simulink model "Gait2392_simbody_simscape"  (R2025b)
(part 2 of 16)

  vas_med_l_vas_med_l_P3_y : sm_lib/Joints/Prismatic Joint  JointMode=Normal  CompositeWrenchDir=FollowerOnBase  CompositeWrenchFrame=BaseFrame  SenseConstraintForce=off  SenseConstraintTorque=off  SenseTotalForce=off  SenseTotalTorque=off  PositionTargetSpecify=off  PositionTargetPriority=High  PositionTargetValue=0  PositionTargetValueUnits=m  VelocityTargetSpecify=off  VelocityTargetPriority=High  VelocityTargetValue=0  VelocityTargetValueUnits=m/s  EquilibriumPosition=0  EquilibriumPositionUnits=m  SpringStiffness=0  SpringStiffnessUnits=N/m  DampingCoefficient=0  DampingCoefficientUnits=kg/s  LowerLimitSpecify=on  LowerLimitBound=-0.4048  LowerLimitBoundUnits=m  LowerLimitStiffness=1e6  LowerLimitStiffnessUnits=N/m  LowerLimitDamping=1e3  LowerLimitDampingUnits=N/(m/s)  LowerLimitTransitionRegionWidth=1e-4  LowerLimitTransitionRegionWidthUnits=m  UpperLimitSpecify=on  UpperLimitBound=-0.2769  UpperLimitBoundUnits=m  UpperLimitStiffness=1e6  UpperLimitStiffnessUnits=N/m  UpperLimitDamping=1e3  UpperLimitDampingUnits=N/(m/s)  UpperLimitTransitionRegionWidth=1e-4  UpperLimitTransitionRegionWidthUnits=m  TorqueActuationMode=NoTorque  MotionActuationMode=ComputedMotion  SensePosition=off  SenseVelocity=off  SenseAcceleration=off  SenseTorqueForce=off  SenseLowerLimitTorqueForce=off  SenseUpperLimitTorqueForce=off
  vas_med_l_vas_med_l_P3_z : sm_lib/Joints/Prismatic Joint  JointMode=Normal  CompositeWrenchDir=FollowerOnBase  CompositeWrenchFrame=BaseFrame  SenseConstraintForce=off  SenseConstraintTorque=off  SenseTotalForce=off  SenseTotalTorque=off  PositionTargetSpecify=off  PositionTargetPriority=High  PositionTargetValue=0  PositionTargetValueUnits=m  VelocityTargetSpecify=off  VelocityTargetPriority=High  VelocityTargetValue=0  VelocityTargetValueUnits=m/s  EquilibriumPosition=0  EquilibriumPositionUnits=m  SpringStiffness=0  SpringStiffnessUnits=N/m  DampingCoefficient=0  DampingCoefficientUnits=kg/s  LowerLimitSpecify=on  LowerLimitBound=-0.0009  LowerLimitBoundUnits=m  LowerLimitStiffness=1e6  LowerLimitStiffnessUnits=N/m  LowerLimitDamping=1e3  LowerLimitDampingUnits=N/(m/s)  LowerLimitTransitionRegionWidth=1e-4  LowerLimitTransitionRegionWidthUnits=m  UpperLimitSpecify=on  UpperLimitBound=0.0125  UpperLimitBoundUnits=m  UpperLimitStiffness=1e6  UpperLimitStiffnessUnits=N/m  UpperLimitDamping=1e3  UpperLimitDampingUnits=N/(m/s)  UpperLimitTransitionRegionWidth=1e-4  UpperLimitTransitionRegionWidthUnits=m  TorqueActuationMode=NoTorque  MotionActuationMode=ComputedMotion  SensePosition=off  SenseVelocity=off  SenseAcceleration=off  SenseTorqueForce=off  SenseLowerLimitTorqueForce=off  SenseUpperLimitTorqueForce=off
  vas_med_l_vas_med_l_P4 : Subsystem
  vas_med_l_vas_med_l_P4_frame_fix : sm_lib/Joints/Weld Joint  JointMode=Normal  CompositeWrenchDir=FollowerOnBase  CompositeWrenchFrame=BaseFrame  SenseConstraintForce=off  SenseConstraintTorque=off  SenseTotalForce=off  SenseTotalTorque=off
  vas_med_l_vas_med_l_P4_vas_med_l_vas_med_l_P4_x_f : Subsystem
  vas_med_l_vas_med_l_P4_vas_med_l_vas_med_l_P4_y_f : Subsystem
  vas_med_l_vas_med_l_P4_vas_med_l_vas_med_l_P4_z_f : Subsystem
  vas_med_l_vas_med_l_P4_x : sm_lib/Joints/Prismatic Joint  JointMode=Normal  CompositeWrenchDir=FollowerOnBase  CompositeWrenchFrame=BaseFrame  SenseConstraintForce=off  SenseConstraintTorque=off  SenseTotalForce=off  SenseTotalTorque=off  PositionTargetSpecify=off  PositionTargetPriority=High  PositionTargetValue=0  PositionTargetValueUnits=m  VelocityTargetSpecify=off  VelocityTargetPriority=High  VelocityTargetValue=0  VelocityTargetValueUnits=m/s  EquilibriumPosition=0  EquilibriumPositionUnits=m  SpringStiffness=0  SpringStiffnessUnits=N/m  DampingCoefficient=0  DampingCoefficientUnits=kg/s  LowerLimitSpecify=on  LowerLimitBound=0.0274  LowerLimitBoundUnits=m  LowerLimitStiffness=1e6  LowerLimitStiffnessUnits=N/m  LowerLimitDamping=1e3  LowerLimitDampingUnits=N/(m/s)  LowerLimitTransitionRegionWidth=1e-4  LowerLimitTransitionRegionWidthUnits=m  UpperLimitSpecify=on  UpperLimitBound=0.0356  UpperLimitBoundUnits=m  UpperLimitStiffness=1e6  UpperLimitStiffnessUnits=N/m  UpperLimitDamping=1e3  UpperLimitDampingUnits=N/(m/s)  UpperLimitTransitionRegionWidth=1e-4  UpperLimitTransitionRegionWidthUnits=m  TorqueActuationMode=NoTorque  MotionActuationMode=ComputedMotion  SensePosition=off  SenseVelocity=off  SenseAcceleration=off  SenseTorqueForce=off  SenseLowerLimitTorqueForce=off  SenseUpperLimitTorqueForce=off
  vas_med_l_vas_med_l_P4_y : sm_lib/Joints/Prismatic Joint  JointMode=Normal  CompositeWrenchDir=FollowerOnBase  CompositeWrenchFrame=BaseFrame  SenseConstraintForce=off  SenseConstraintTorque=off  SenseTotalForce=off  SenseTotalTorque=off  PositionTargetSpecify=off  PositionTargetPriority=High  PositionTargetValue=0  PositionTargetValueUnits=m  VelocityTargetSpecify=off  VelocityTargetPriority=High  VelocityTargetValue=0  VelocityTargetValueUnits=m/s  EquilibriumPosition=0  EquilibriumPositionUnits=m  SpringStiffness=0  SpringStiffnessUnits=N/m  DampingCoefficient=0  DampingCoefficientUnits=kg/s  LowerLimitSpecify=on  LowerLimitBound=-0.4255  LowerLimitBoundUnits=m  LowerLimitStiffness=1e6  LowerLimitStiffnessUnits=N/m  LowerLimitDamping=1e3  LowerLimitDampingUnits=N/(m/s)  LowerLimitTransitionRegionWidth=1e-4  LowerLimitTransitionRegionWidthUnits=m  UpperLimitSpecify=on  UpperLimitBound=-0.2769  UpperLimitBoundUnits=m  UpperLimitStiffness=1e6  UpperLimitStiffnessUnits=N/m  UpperLimitDamping=1e3  UpperLimitDampingUnits=N/(m/s)  UpperLimitTransitionRegionWidth=1e-4  UpperLimitTransitionRegionWidthUnits=m  TorqueActuationMode=NoTorque  MotionActuationMode=ComputedMotion  SensePosition=off  SenseVelocity=off  SenseAcceleration=off  SenseTorqueForce=off  SenseLowerLimitTorqueForce=off  SenseUpperLimitTorqueForce=off
  vas_med_l_vas_med_l_P4_z : sm_lib/Joints/Prismatic Joint  JointMode=Normal  CompositeWrenchDir=FollowerOnBase  CompositeWrenchFrame=BaseFrame  SenseConstraintForce=off  SenseConstraintTorque=off  SenseTotalForce=off  SenseTotalTorque=off  PositionTargetSpecify=off  PositionTargetPriority=High  PositionTargetValue=0  PositionTargetValueUnits=m  VelocityTargetSpecify=off  VelocityTargetPriority=High  VelocityTargetValue=0  VelocityTargetValueUnits=m/s  EquilibriumPosition=0  EquilibriumPositionUnits=m  SpringStiffness=0  SpringStiffnessUnits=N/m  DampingCoefficient=0  DampingCoefficientUnits=kg/s  LowerLimitSpecify=on  LowerLimitBound=-0.0009  LowerLimitBoundUnits=m  LowerLimitStiffness=1e6  LowerLimitStiffnessUnits=N/m  LowerLimitDamping=1e3  LowerLimitDampingUnits=N/(m/s)  LowerLimitTransitionRegionWidth=1e-4  LowerLimitTransitionRegionWidthUnits=m  UpperLimitSpecify=on  UpperLimitBound=0.0131  UpperLimitBoundUnits=m  UpperLimitStiffness=1e6  UpperLimitStiffnessUnits=N/m  UpperLimitDamping=1e3  UpperLimitDampingUnits=N/(m/s)  UpperLimitTransitionRegionWidth=1e-4  UpperLimitTransitionRegionWidthUnits=m  TorqueActuationMode=NoTorque  MotionActuationMode=ComputedMotion  SensePosition=off  SenseVelocity=off  SenseAcceleration=off  SenseTorqueForce=off  SenseLowerLimitTorqueForce=off  SenseUpperLimitTorqueForce=off
  vas_med_l_vas_med_l_P5 : Subsystem
  vas_med_l_vas_med_l_P5_frame_fix : sm_lib/Joints/Weld Joint  JointMode=Normal  CompositeWrenchDir=FollowerOnBase  CompositeWrenchFrame=BaseFrame  SenseConstraintForce=off  SenseConstraintTorque=off  SenseTotalForce=off  SenseTotalTorque=off
  vas_med_l_vas_med_l_P5_vas_med_l_vas_med_l_P5_x_f : Subsystem
  vas_med_l_vas_med_l_P5_vas_med_l_vas_med_l_P5_y_f : Subsystem
  vas_med_l_vas_med_l_P5_x : sm_lib/Joints/Prismatic Joint  JointMode=Normal  CompositeWrenchDir=FollowerOnBase  CompositeWrenchFrame=BaseFrame  SenseConstraintForce=off  SenseConstraintTorque=off  SenseTotalForce=off  SenseTotalTorque=off  PositionTargetSpecify=off  PositionTargetPriority=High  PositionTargetValue=0  PositionTargetValueUnits=m  VelocityTargetSpecify=off  VelocityTargetPriority=High  VelocityTargetValue=0  VelocityTargetValueUnits=m/s  EquilibriumPosition=0  EquilibriumPositionUnits=m  SpringStiffness=0  SpringStiffnessUnits=N/m  DampingCoefficient=0  DampingCoefficientUnits=kg/s  LowerLimitSpecify=on  LowerLimitBound=0.009811  LowerLimitBoundUnits=m  LowerLimitStiffness=1e6  LowerLimitStiffnessUnits=N/m  LowerLimitDamping=1e3  LowerLimitDampingUnits=N/(m/s)  LowerLimitTransitionRegionWidth=1e-4  LowerLimitTransitionRegionWidthUnits=m  UpperLimitSpecify=on  UpperLimitBound=0.06795  UpperLimitBoundUnits=m  UpperLimitStiffness=1e6  UpperLimitStiffnessUnits=N/m  UpperLimitDamping=1e3  UpperLimitDampingUnits=N/(m/s)  UpperLimitTransitionRegionWidth=1e-4  UpperLimitTransitionRegionWidthUnits=m  TorqueActuationMode=NoTorque  MotionActuationMode=ComputedMotion  SensePosition=off  SenseVelocity=off  SenseAcceleration=off  SenseTorqueForce=off  SenseLowerLimitTorqueForce=off  SenseUpperLimitTorqueForce=off
  vas_med_l_vas_med_l_P5_y : sm_lib/Joints/Prismatic Joint  JointMode=Normal  CompositeWrenchDir=FollowerOnBase  CompositeWrenchFrame=BaseFrame  SenseConstraintForce=off  SenseConstraintTorque=off  SenseTotalForce=off  SenseTotalTorque=off  PositionTargetSpecify=off  PositionTargetPriority=High  PositionTargetValue=0  PositionTargetValueUnits=m  VelocityTargetSpecify=off  VelocityTargetPriority=High  VelocityTargetValue=0  VelocityTargetValueUnits=m/s  EquilibriumPosition=0  EquilibriumPositionUnits=m  SpringStiffness=0  SpringStiffnessUnits=N/m  DampingCoefficient=0  DampingCoefficientUnits=kg/s  LowerLimitSpecify=on  LowerLimitBound=-0.06562  LowerLimitBoundUnits=m  LowerLimitStiffness=1e6  LowerLimitStiffnessUnits=N/m  LowerLimitDamping=1e3  LowerLimitDampingUnits=N/(m/s)  LowerLimitTransitionRegionWidth=1e-4  LowerLimitTransitionRegionWidthUnits=m  UpperLimitSpecify=on  UpperLimitBound=0.02433  UpperLimitBoundUnits=m  UpperLimitStiffness=1e6  UpperLimitStiffnessUnits=N/m  UpperLimitDamping=1e3  UpperLimitDampingUnits=N/(m/s)  UpperLimitTransitionRegionWidth=1e-4  UpperLimitTransitionRegionWidthUnits=m  TorqueActuationMode=NoTorque  MotionActuationMode=ComputedMotion  SensePosition=off  SenseVelocity=off  SenseAcceleration=off  SenseTorqueForce=off  SenseLowerLimitTorqueForce=off  SenseUpperLimitTorqueForce=off
  vas_med_r_vas_med_r_P3 : Subsystem
  vas_med_r_vas_med_r_P3_frame_fix : sm_lib/Joints/Weld Joint  JointMode=Normal  CompositeWrenchDir=FollowerOnBase  CompositeWrenchFrame=BaseFrame  SenseConstraintForce=off  SenseConstraintTorque=off  SenseTotalForce=off  SenseTotalTorque=off
  vas_med_r_vas_med_r_P3_vas_med_r_vas_med_r_P3_x_f : Subsystem
  vas_med_r_vas_med_r_P3_vas_med_r_vas_med_r_P3_y_f : Subsystem
  vas_med_r_vas_med_r_P3_vas_med_r_vas_med_r_P3_z_f : Subsystem
  vas_med_r_vas_med_r_P3_x : sm_lib/Joints/Prismatic Joint  JointMode=Normal  CompositeWrenchDir=FollowerOnBase  CompositeWrenchFrame=BaseFrame  SenseConstraintForce=off  SenseConstraintTorque=off  SenseTotalForce=off  SenseTotalTorque=off  PositionTargetSpecify=off  PositionTargetPriority=High  PositionTargetValue=0  PositionTargetValueUnits=m  VelocityTargetSpecify=off  VelocityTargetPriority=High  VelocityTargetValue=0  VelocityTargetValueUnits=m/s  EquilibriumPosition=0  EquilibriumPositionUnits=m  SpringStiffness=0  SpringStiffnessUnits=N/m  DampingCoefficient=0  DampingCoefficientUnits=kg/s  LowerLimitSpecify=on  LowerLimitBound=0.0356  LowerLimitBoundUnits=m  LowerLimitStiffness=1e6  LowerLimitStiffnessUnits=N/m  LowerLimitDamping=1e3  LowerLimitDampingUnits=N/(m/s)  LowerLimitTransitionRegionWidth=1e-4  LowerLimitTransitionRegionWidthUnits=m  UpperLimitSpecify=on  UpperLimitBound=0.037  UpperLimitBoundUnits=m  UpperLimitStiffness=1e6  UpperLimitStiffnessUnits=N/m  UpperLimitDamping=1e3  UpperLimitDampingUnits=N/(m/s)  UpperLimitTransitionRegionWidth=1e-4  UpperLimitTransitionRegionWidthUnits=m  TorqueActuationMode=NoTorque  MotionActuationMode=ComputedMotion  SensePosition=off  SenseVelocity=off  SenseAcceleration=off  SenseTorqueForce=off  SenseLowerLimitTorqueForce=off  SenseUpperLimitTorqueForce=off
  vas_med_r_vas_med_r_P3_y : sm_lib/Joints/Prismatic Joint  JointMode=Normal  CompositeWrenchDir=FollowerOnBase  CompositeWrenchFrame=BaseFrame  SenseConstraintForce=off  SenseConstraintTorque=off  SenseTotalForce=off  SenseTotalTorque=off  PositionTargetSpecify=off  PositionTargetPriority=High  PositionTargetValue=0  PositionTargetValueUnits=m  VelocityTargetSpecify=off  VelocityTargetPriority=High  VelocityTargetValue=0  VelocityTargetValueUnits=m/s  EquilibriumPosition=0  EquilibriumPositionUnits=m  SpringStiffness=0  SpringStiffnessUnits=N/m  DampingCoefficient=0  DampingCoefficientUnits=kg/s  LowerLimitSpecify=on  LowerLimitBound=-0.4048  LowerLimitBoundUnits=m  LowerLimitStiffness=1e6  LowerLimitStiffnessUnits=N/m  LowerLimitDamping=1e3  LowerLimitDampingUnits=N/(m/s)  LowerLimitTransitionRegionWidth=1e-4  LowerLimitTransitionRegionWidthUnits=m  UpperLimitSpecify=on  UpperLimitBound=-0.2769  UpperLimitBoundUnits=m  UpperLimitStiffness=1e6  UpperLimitStiffnessUnits=N/m  UpperLimitDamping=1e3  UpperLimitDampingUnits=N/(m/s)  UpperLimitTransitionRegionWidth=1e-4  UpperLimitTransitionRegionWidthUnits=m  TorqueActuationMode=NoTorque  MotionActuationMode=ComputedMotion  SensePosition=off  SenseVelocity=off  SenseAcceleration=off  SenseTorqueForce=off  SenseLowerLimitTorqueForce=off  SenseUpperLimitTorqueForce=off
  vas_med_r_vas_med_r_P3_z : sm_lib/Joints/Prismatic Joint  JointMode=Normal  CompositeWrenchDir=FollowerOnBase  CompositeWrenchFrame=BaseFrame  SenseConstraintForce=off  SenseConstraintTorque=off  SenseTotalForce=off  SenseTotalTorque=off  PositionTargetSpecify=off  PositionTargetPriority=High  PositionTargetValue=0  PositionTargetValueUnits=m  VelocityTargetSpecify=off  VelocityTargetPriority=High  VelocityTargetValue=0  VelocityTargetValueUnits=m/s  EquilibriumPosition=0  EquilibriumPositionUnits=m  SpringStiffness=0  SpringStiffnessUnits=N/m  DampingCoefficient=0  DampingCoefficientUnits=kg/s  LowerLimitSpecify=on  LowerLimitBound=-0.0125  LowerLimitBoundUnits=m  LowerLimitStiffness=1e6  LowerLimitStiffnessUnits=N/m  LowerLimitDamping=1e3  LowerLimitDampingUnits=N/(m/s)  LowerLimitTransitionRegionWidth=1e-4  LowerLimitTransitionRegionWidthUnits=m  UpperLimitSpecify=on  UpperLimitBound=0.0009  UpperLimitBoundUnits=m  UpperLimitStiffness=1e6  UpperLimitStiffnessUnits=N/m  UpperLimitDamping=1e3  UpperLimitDampingUnits=N/(m/s)  UpperLimitTransitionRegionWidth=1e-4  UpperLimitTransitionRegionWidthUnits=m  TorqueActuationMode=NoTorque  MotionActuationMode=ComputedMotion  SensePosition=off  SenseVelocity=off  SenseAcceleration=off  SenseTorqueForce=off  SenseLowerLimitTorqueForce=off  SenseUpperLimitTorqueForce=off
  vas_med_r_vas_med_r_P4 : Subsystem
  vas_med_r_vas_med_r_P4_frame_fix : sm_lib/Joints/Weld Joint  JointMode=Normal  CompositeWrenchDir=FollowerOnBase  CompositeWrenchFrame=BaseFrame  SenseConstraintForce=off  SenseConstraintTorque=off  SenseTotalForce=off  SenseTotalTorque=off
  vas_med_r_vas_med_r_P4_vas_med_r_vas_med_r_P4_x_f : Subsystem
  vas_med_r_vas_med_r_P4_vas_med_r_vas_med_r_P4_y_f : Subsystem
  vas_med_r_vas_med_r_P4_vas_med_r_vas_med_r_P4_z_f : Subsystem
  vas_med_r_vas_med_r_P4_x : sm_lib/Joints/Prismatic Joint  JointMode=Normal  CompositeWrenchDir=FollowerOnBase  CompositeWrenchFrame=BaseFrame  SenseConstraintForce=off  SenseConstraintTorque=off  SenseTotalForce=off  SenseTotalTorque=off  PositionTargetSpecify=off  PositionTargetPriority=High  PositionTargetValue=0  PositionTargetValueUnits=m  VelocityTargetSpecify=off  VelocityTargetPriority=High  VelocityTargetValue=0  VelocityTargetValueUnits=m/s  EquilibriumPosition=0  EquilibriumPositionUnits=m  SpringStiffness=0  SpringStiffnessUnits=N/m  DampingCoefficient=0  DampingCoefficientUnits=kg/s  LowerLimitSpecify=on  LowerLimitBound=0.0274  LowerLimitBoundUnits=m  LowerLimitStiffness=1e6  LowerLimitStiffnessUnits=N/m  LowerLimitDamping=1e3  LowerLimitDampingUnits=N/(m/s)  LowerLimitTransitionRegionWidth=1e-4  LowerLimitTransitionRegionWidthUnits=m  UpperLimitSpecify=on  UpperLimitBound=0.0356  UpperLimitBoundUnits=m  UpperLimitStiffness=1e6  UpperLimitStiffnessUnits=N/m  UpperLimitDamping=1e3  UpperLimitDampingUnits=N/(m/s)  UpperLimitTransitionRegionWidth=1e-4  UpperLimitTransitionRegionWidthUnits=m  TorqueActuationMode=NoTorque  MotionActuationMode=ComputedMotion  SensePosition=off  SenseVelocity=off  SenseAcceleration=off  SenseTorqueForce=off  SenseLowerLimitTorqueForce=off  SenseUpperLimitTorqueForce=off
  vas_med_r_vas_med_r_P4_y : sm_lib/Joints/Prismatic Joint  JointMode=Normal  CompositeWrenchDir=FollowerOnBase  CompositeWrenchFrame=BaseFrame  SenseConstraintForce=off  SenseConstraintTorque=off  SenseTotalForce=off  SenseTotalTorque=off  PositionTargetSpecify=off  PositionTargetPriority=High  PositionTargetValue=0  PositionTargetValueUnits=m  VelocityTargetSpecify=off  VelocityTargetPriority=High  VelocityTargetValue=0  VelocityTargetValueUnits=m/s  EquilibriumPosition=0  EquilibriumPositionUnits=m  SpringStiffness=0  SpringStiffnessUnits=N/m  DampingCoefficient=0  DampingCoefficientUnits=kg/s  LowerLimitSpecify=on  LowerLimitBound=-0.4255  LowerLimitBoundUnits=m  LowerLimitStiffness=1e6  LowerLimitStiffnessUnits=N/m  LowerLimitDamping=1e3  LowerLimitDampingUnits=N/(m/s)  LowerLimitTransitionRegionWidth=1e-4  LowerLimitTransitionRegionWidthUnits=m  UpperLimitSpecify=on  UpperLimitBound=-0.2769  UpperLimitBoundUnits=m  UpperLimitStiffness=1e6  UpperLimitStiffnessUnits=N/m  UpperLimitDamping=1e3  UpperLimitDampingUnits=N/(m/s)  UpperLimitTransitionRegionWidth=1e-4  UpperLimitTransitionRegionWidthUnits=m  TorqueActuationMode=NoTorque  MotionActuationMode=ComputedMotion  SensePosition=off  SenseVelocity=off  SenseAcceleration=off  SenseTorqueForce=off  SenseLowerLimitTorqueForce=off  SenseUpperLimitTorqueForce=off
  vas_med_r_vas_med_r_P4_z : sm_lib/Joints/Prismatic Joint  JointMode=Normal  CompositeWrenchDir=FollowerOnBase  CompositeWrenchFrame=BaseFrame  SenseConstraintForce=off  SenseConstraintTorque=off  SenseTotalForce=off  SenseTotalTorque=off  PositionTargetSpecify=off  PositionTargetPriority=High  PositionTargetValue=0  PositionTargetValueUnits=m  VelocityTargetSpecify=off  VelocityTargetPriority=High  VelocityTargetValue=0  VelocityTargetValueUnits=m/s  EquilibriumPosition=0  EquilibriumPositionUnits=m  SpringStiffness=0  SpringStiffnessUnits=N/m  DampingCoefficient=0  DampingCoefficientUnits=kg/s  LowerLimitSpecify=on  LowerLimitBound=-0.0131  LowerLimitBoundUnits=m  LowerLimitStiffness=1e6  LowerLimitStiffnessUnits=N/m  LowerLimitDamping=1e3  LowerLimitDampingUnits=N/(m/s)  LowerLimitTransitionRegionWidth=1e-4  LowerLimitTransitionRegionWidthUnits=m  UpperLimitSpecify=on  UpperLimitBound=0.0009  UpperLimitBoundUnits=m  UpperLimitStiffness=1e6  UpperLimitStiffnessUnits=N/m  UpperLimitDamping=1e3  UpperLimitDampingUnits=N/(m/s)  UpperLimitTransitionRegionWidth=1e-4  UpperLimitTransitionRegionWidthUnits=m  TorqueActuationMode=NoTorque  MotionActuationMode=ComputedMotion  SensePosition=off  SenseVelocity=off  SenseAcceleration=off  SenseTorqueForce=off  SenseLowerLimitTorqueForce=off  SenseUpperLimitTorqueForce=off
  vas_med_r_vas_med_r_P5 : Subsystem
  vas_med_r_vas_med_r_P5_frame_fix : sm_lib/Joints/Weld Joint  JointMode=Normal  CompositeWrenchDir=FollowerOnBase  CompositeWrenchFrame=BaseFrame  SenseConstraintForce=off  SenseConstraintTorque=off  SenseTotalForce=off  SenseTotalTorque=off
  vas_med_r_vas_med_r_P5_vas_med_r_vas_med_r_P5_x_f : Subsystem
  vas_med_r_vas_med_r_P5_vas_med_r_vas_med_r_P5_y_f : Subsystem
  vas_med_r_vas_med_r_P5_x : sm_lib/Joints/Prismatic Joint  JointMode=Normal  CompositeWrenchDir=FollowerOnBase  CompositeWrenchFrame=BaseFrame  SenseConstraintForce=off  SenseConstraintTorque=off  SenseTotalForce=off  SenseTotalTorque=off  PositionTargetSpecify=off  PositionTargetPriority=High  PositionTargetValue=0  PositionTargetValueUnits=m  VelocityTargetSpecify=off  VelocityTargetPriority=High  VelocityTargetValue=0  VelocityTargetValueUnits=m/s  EquilibriumPosition=0  EquilibriumPositionUnits=m  SpringStiffness=0  SpringStiffnessUnits=N/m  DampingCoefficient=0  DampingCoefficientUnits=kg/s  LowerLimitSpecify=on  LowerLimitBound=0.009811  LowerLimitBoundUnits=m  LowerLimitStiffness=1e6  LowerLimitStiffnessUnits=N/m  LowerLimitDamping=1e3  LowerLimitDampingUnits=N/(m/s)  LowerLimitTransitionRegionWidth=1e-4  LowerLimitTransitionRegionWidthUnits=m  UpperLimitSpecify=on  UpperLimitBound=0.06795  UpperLimitBoundUnits=m  UpperLimitStiffness=1e6  UpperLimitStiffnessUnits=N/m  UpperLimitDamping=1e3  UpperLimitDampingUnits=N/(m/s)  UpperLimitTransitionRegionWidth=1e-4  UpperLimitTransitionRegionWidthUnits=m  TorqueActuationMode=NoTorque  MotionActuationMode=ComputedMotion  SensePosition=off  SenseVelocity=off  SenseAcceleration=off  SenseTorqueForce=off  SenseLowerLimitTorqueForce=off  SenseUpperLimitTorqueForce=off
  vas_med_r_vas_med_r_P5_y : sm_lib/Joints/Prismatic Joint  JointMode=Normal  CompositeWrenchDir=FollowerOnBase  CompositeWrenchFrame=BaseFrame  SenseConstraintForce=off  SenseConstraintTorque=off  SenseTotalForce=off  SenseTotalTorque=off  PositionTargetSpecify=off  PositionTargetPriority=High  PositionTargetValue=0  PositionTargetValueUnits=m  VelocityTargetSpecify=off  VelocityTargetPriority=High  VelocityTargetValue=0  VelocityTargetValueUnits=m/s  EquilibriumPosition=0  EquilibriumPositionUnits=m  SpringStiffness=0  SpringStiffnessUnits=N/m  DampingCoefficient=0  DampingCoefficientUnits=kg/s  LowerLimitSpecify=on  LowerLimitBound=-0.06562  LowerLimitBoundUnits=m  LowerLimitStiffness=1e6  LowerLimitStiffnessUnits=N/m  LowerLimitDamping=1e3  LowerLimitDampingUnits=N/(m/s)  LowerLimitTransitionRegionWidth=1e-4  LowerLimitTransitionRegionWidthUnits=m  UpperLimitSpecify=on  UpperLimitBound=0.02433  UpperLimitBoundUnits=m  UpperLimitStiffness=1e6  UpperLimitStiffnessUnits=N/m  UpperLimitDamping=1e3  UpperLimitDampingUnits=N/(m/s)  UpperLimitTransitionRegionWidth=1e-4  UpperLimitTransitionRegionWidthUnits=m  TorqueActuationMode=NoTorque  MotionActuationMode=ComputedMotion  SensePosition=off  SenseVelocity=off  SenseAcceleration=off  SenseTorqueForce=off  SenseLowerLimitTorqueForce=off  SenseUpperLimitTorqueForce=off
  world : Subsystem
  connections:
  calcn_l/LConn1 -- calcn_l_frame_fix/RConn1
  calcn_l/RConn1 -- mtp_angle_l/LConn1
  femur_l/RConn7 -- lat_gas_l_lat_gas_l_P2_x/LConn1
  pelvis_pelvis_tx_f/LConn1 -- pelvis_tx/RConn1
  pelvis_pelvis_tx_f/RConn1 -- pelvis_ty/LConn1
  pelvis_pelvis_ty_f/LConn1 -- pelvis_ty/RConn1
  pelvis_pelvis_ty_f/RConn1 -- pelvis_tz/LConn1
  pelvis_pelvis_tz_f/LConn1 -- pelvis_tz/RConn1
  pelvis_pelvis_tz_f/RConn1 -- pelvis_tilt/LConn1
  psoas_l_psoas_l_P3/LConn1 -- psoas_l_psoas_l_P3_frame_fix/RConn1
  psoas_l_psoas_l_P3_psoas_l_psoas_l_P3_x_f/LConn1 -- psoas_l_psoas_l_P3_x/RConn1
  psoas_l_psoas_l_P3_psoas_l_psoas_l_P3_x_f/RConn1 -- psoas_l_psoas_l_P3_y/LConn1
  psoas_l_psoas_l_P3_psoas_l_psoas_l_P3_y_f/LConn1 -- psoas_l_psoas_l_P3_y/RConn1
  femur_l/RConn6 -- med_gas_l_med_gas_l_P2_x/LConn1
  psoas_l_psoas_l_P3_psoas_l_psoas_l_P3_y_f/RConn1 -- psoas_l_psoas_l_P3_z/LConn1
  psoas_l_psoas_l_P3_psoas_l_psoas_l_P3_z_f/LConn1 -- psoas_l_psoas_l_P3_z/RConn1
  psoas_l_psoas_l_P3_frame_fix/LConn1 -- psoas_l_psoas_l_P3_psoas_l_psoas_l_P3_z_f/RConn1
  psoas_r_psoas_r_P3/LConn1 -- psoas_r_psoas_r_P3_frame_fix/RConn1
  psoas_r_psoas_r_P3_psoas_r_psoas_r_P3_x_f/LConn1 -- psoas_r_psoas_r_P3_x/RConn1
  psoas_r_psoas_r_P3_psoas_r_psoas_r_P3_x_f/RConn1 -- psoas_r_psoas_r_P3_y/LConn1
  psoas_r_psoas_r_P3_psoas_r_psoas_r_P3_y_f/LConn1 -- psoas_r_psoas_r_P3_y/RConn1
  psoas_r_psoas_r_P3_psoas_r_psoas_r_P3_y_f/RConn1 -- psoas_r_psoas_r_P3_z/LConn1
  psoas_r_psoas_r_P3_psoas_r_psoas_r_P3_z_f/LConn1 -- psoas_r_psoas_r_P3_z/RConn1
  psoas_r_psoas_r_P3_frame_fix/LConn1 -- psoas_r_psoas_r_P3_psoas_r_psoas_r_P3_z_f/RConn1
  femur_l/RConn5 -- vas_int_l_vas_int_l_P3_y/LConn1
  rect_fem_l_rect_fem_l_P3/LConn1 -- rect_fem_l_rect_fem_l_P3_frame_fix/RConn1
  rect_fem_l_rect_fem_l_P3_rect_fem_l_rect_fem_l_P3_x_f/LConn1 -- rect_fem_l_rect_fem_l_P3_x/RConn1
  rect_fem_l_rect_fem_l_P3_rect_fem_l_rect_fem_l_P3_x_f/RConn1 -- rect_fem_l_rect_fem_l_P3_y/LConn1
  rect_fem_l_rect_fem_l_P3_rect_fem_l_rect_fem_l_P3_y_f/LConn1 -- rect_fem_l_rect_fem_l_P3_y/RConn1
  rect_fem_l_rect_fem_l_P3_frame_fix/LConn1 -- rect_fem_l_rect_fem_l_P3_rect_fem_l_rect_fem_l_P3_y_f/RConn1
  rect_fem_r_rect_fem_r_P3/LConn1 -- rect_fem_r_rect_fem_r_P3_frame_fix/RConn1
  rect_fem_r_rect_fem_r_P3_rect_fem_r_rect_fem_r_P3_x_f/LConn1 -- rect_fem_r_rect_fem_r_P3_x/RConn1
  rect_fem_r_rect_fem_r_P3_rect_fem_r_rect_fem_r_P3_x_f/RConn1 -- rect_fem_r_rect_fem_r_P3_y/LConn1
  rect_fem_r_rect_fem_r_P3_rect_fem_r_rect_fem_r_P3_y_f/LConn1 -- rect_fem_r_rect_fem_r_P3_y/RConn1
  rect_fem_r_rect_fem_r_P3_frame_fix/LConn1 -- rect_fem_r_rect_fem_r_P3_rect_fem_r_rect_fem_r_P3_y_f/RConn1
  femur_l/RConn4 -- vas_lat_l_vas_lat_l_P3_x/LConn1
  semimem_l_semimem_l_P2/LConn1 -- semimem_l_semimem_l_P2_frame_fix/RConn1
  semimem_l_semimem_l_P2_semimem_l_semimem_l_P2_x_f/LConn1 -- semimem_l_semimem_l_P2_x/RConn1
  semimem_l_semimem_l_P2_semimem_l_semimem_l_P2_x_f/RConn1 -- semimem_l_semimem_l_P2_y/LConn1
  semimem_l_semimem_l_P2_semimem_l_semimem_l_P2_y_f/LConn1 -- semimem_l_semimem_l_P2_y/RConn1
  semimem_l_semimem_l_P2_frame_fix/LConn1 -- semimem_l_semimem_l_P2_semimem_l_semimem_l_P2_y_f/RConn1
  semimem_r_semimem_r_P2/LConn1 -- semimem_r_semimem_r_P2_frame_fix/RConn1
  semimem_r_semimem_r_P2_semimem_r_semimem_r_P2_x_f/LConn1 -- semimem_r_semimem_r_P2_x/RConn1
  semimem_r_semimem_r_P2_semimem_r_semimem_r_P2_x_f/RConn1 -- semimem_r_semimem_r_P2_y/LConn1
  semimem_r_semimem_r_P2_semimem_r_semimem_r_P2_y_f/LConn1 -- semimem_r_semimem_r_P2_y/RConn1
  semimem_r_semimem_r_P2_frame_fix/LConn1 -- semimem_r_semimem_r_P2_semimem_r_semimem_r_P2_y_f/RConn1
  femur_l/RConn3 -- vas_lat_l_vas_lat_l_P4_x/LConn1
  semiten_l_semiten_l_P2/LConn1 -- semiten_l_semiten_l_P2_frame_fix/RConn1
  semiten_l_semiten_l_P2_semiten_l_semiten_l_P2_x_f/LConn1 -- semiten_l_semiten_l_P2_x/RConn1
  semiten_l_semiten_l_P2_semiten_l_semiten_l_P2_x_f/RConn1 -- semiten_l_semiten_l_P2_y/LConn1
  semiten_l_semiten_l_P2_semiten_l_semiten_l_P2_y_f/LConn1 -- semiten_l_semiten_l_P2_y/RConn1
  semiten_l_semiten_l_P2_frame_fix/LConn1 -- semiten_l_semiten_l_P2_semiten_l_semiten_l_P2_y_f/RConn1
  semiten_r_semiten_r_P2/LConn1 -- semiten_r_semiten_r_P2_frame_fix/RConn1
  semiten_r_semiten_r_P2_semiten_r_semiten_r_P2_x_f/LConn1 -- semiten_r_semiten_r_P2_x/RConn1
  semiten_r_semiten_r_P2_semiten_r_semiten_r_P2_x_f/RConn1 -- semiten_r_semiten_r_P2_y/LConn1
  semiten_r_semiten_r_P2_semiten_r_semiten_r_P2_y_f/LConn1 -- semiten_r_semiten_r_P2_y/RConn1
  semiten_r_semiten_r_P2_frame_fix/LConn1 -- semiten_r_semiten_r_P2_semiten_r_semiten_r_P2_y_f/RConn1
  femur_l/RConn2 -- vas_med_l_vas_med_l_P3_x/LConn1
  talus_l/LConn1 -- talus_l_frame_fix/RConn1
  subtalar_angle_l/LConn1 -- talus_l/RConn1
  ankle_angle_l/RConn1 -- talus_l_ankle_angle_l_f/LConn1
  talus_l_ankle_angle_l_f/RConn1 -- talus_l_frame_fix/LConn1
  talus_r/LConn1 -- talus_r_frame_fix/RConn1
  subtalar_angle_r/LConn1 -- talus_r/RConn1
  ankle_angle_r/RConn1 -- talus_r_ankle_angle_r_f/LConn1
  talus_r_ankle_angle_r_f/RConn1 -- talus_r_frame_fix/LConn1
  tibia_l/LConn1 -- tibia_l_frame_fix/RConn1
  ankle_angle_l/LConn1 -- tibia_l/RConn8
  femur_l/RConn1 -- vas_med_l_vas_med_l_P4_x/LConn1
  grac_l_grac_l_P2_x/LConn1 -- tibia_l/RConn7
  rect_fem_l_rect_fem_l_P3_x/LConn1 -- tibia_l/RConn6
  semimem_l_semimem_l_P2_x/LConn1 -- tibia_l/RConn5
  semiten_l_semiten_l_P2_x/LConn1 -- tibia_l/RConn4
  tibia_l/RConn3 -- vas_int_l_vas_int_l_P4_x/LConn1
  tibia_l/RConn2 -- vas_lat_l_vas_lat_l_P5_x/LConn1
  tibia_l/RConn1 -- vas_med_l_vas_med_l_P5_x/LConn1
  knee_angle_l/RConn1 -- tibia_l_knee_angle_l_f/LConn1
  tibia_l_frame_fix/LConn1 -- tibia_l_knee_angle_l_f/RConn1
  knee_l_translation1/RConn1 -- tibia_l_knee_l_translation1_f/LConn1
  femur_l_hip_adduction_l_f/LConn1 -- hip_adduction_l/RConn1
  knee_l_translation2/LConn1 -- tibia_l_knee_l_translation1_f/RConn1
  knee_l_translation2/RConn1 -- tibia_l_knee_l_translation2_f/LConn1
  knee_angle_l/LConn1 -- tibia_l_knee_l_translation2_f/RConn1
  tibia_r/LConn1 -- tibia_r_frame_fix/RConn1
  ankle_angle_r/LConn1 -- tibia_r/RConn8
  grac_r_grac_r_P2_x/LConn1 -- tibia_r/RConn7
  rect_fem_r_rect_fem_r_P3_x/LConn1 -- tibia_r/RConn6
  semimem_r_semimem_r_P2_x/LConn1 -- tibia_r/RConn5
  semiten_r_semiten_r_P2_x/LConn1 -- tibia_r/RConn4
  tibia_r/RConn3 -- vas_int_r_vas_int_r_P4_x/LConn1
  femur_l_hip_adduction_l_f/RConn1 -- hip_rotation_l/LConn1
  tibia_r/RConn2 -- vas_lat_r_vas_lat_r_P5_x/LConn1
  tibia_r/RConn1 -- vas_med_r_vas_med_r_P5_x/LConn1
  knee_angle_r/RConn1 -- tibia_r_knee_angle_r_f/LConn1
  tibia_r_frame_fix/LConn1 -- tibia_r_knee_angle_r_f/RConn1
  knee_r_translation1/RConn1 -- tibia_r_knee_r_translation1_f/LConn1
  knee_r_translation2/LConn1 -- tibia_r_knee_r_translation1_f/RConn1
  knee_r_translation2/RConn1 -- tibia_r_knee_r_translation2_f/LConn1
  knee_angle_r/LConn1 -- tibia_r_knee_r_translation2_f/RConn1
  toes_l/LConn1 -- toes_l_frame_fix/RConn1
  mtp_angle_l/RConn1 -- toes_l_mtp_angle_l_f/LConn1
  femur_l_hip_flexion_l_f/LConn1 -- hip_flexion_l/RConn1
  toes_l_frame_fix/LConn1 -- toes_l_mtp_angle_l_f/RConn1
  toes_r/LConn1 -- toes_r_frame_fix/RConn1
  mtp_angle_r/RConn1 -- toes_r_mtp_angle_r_f/LConn1
  toes_r_frame_fix/LConn1 -- toes_r_mtp_angle_r_f/RConn1
  torso/LConn1 -- torso_frame_fix/RConn1
  lumbar_bending/RConn1 -- torso_lumbar_bending_f/LConn1
  lumbar_rotation/LConn1 -- torso_lumbar_bending_f/RConn1
  lumbar_extension/RConn1 -- torso_lumbar_extension_f/LConn1
  lumbar_bending/LConn1 -- torso_lumbar_extension_f/RConn1
  lumbar_rotation/RConn1 -- torso_lumbar_rotation_f/LConn1
  calcn_l_subtalar_angle_l_f/LConn1 -- subtalar_angle_l/RConn1
  femur_l_hip_flexion_l_f/RConn1 -- hip_adduction_l/LConn1
  torso_frame_fix/LConn1 -- torso_lumbar_rotation_f/RConn1
  vas_int_l_vas_int_l_P3/LConn1 -- vas_int_l_vas_int_l_P3_frame_fix/RConn1
  vas_int_l_vas_int_l_P3_vas_int_l_vas_int_l_P3_y_f/LConn1 -- vas_int_l_vas_int_l_P3_y/RConn1
  vas_int_l_vas_int_l_P3_vas_int_l_vas_int_l_P3_y_f/RConn1 -- vas_int_l_vas_int_l_P3_z/LConn1
  vas_int_l_vas_int_l_P3_vas_int_l_vas_int_l_P3_z_f/LConn1 -- vas_int_l_vas_int_l_P3_z/RConn1
  vas_int_l_vas_int_l_P3_frame_fix/LConn1 -- vas_int_l_vas_int_l_P3_vas_int_l_vas_int_l_P3_z_f/RConn1
  vas_int_l_vas_int_l_P4/LConn1 -- vas_int_l_vas_int_l_P4_frame_fix/RConn1
  vas_int_l_vas_int_l_P4_vas_int_l_vas_int_l_P4_x_f/LConn1 -- vas_int_l_vas_int_l_P4_x/RConn1
  vas_int_l_vas_int_l_P4_vas_int_l_vas_int_l_P4_x_f/RConn1 -- vas_int_l_vas_int_l_P4_y/LConn1
  vas_int_l_vas_int_l_P4_vas_int_l_vas_int_l_P4_y_f/LConn1 -- vas_int_l_vas_int_l_P4_y/RConn1
  femur_l_hip_rotation_l_f/LConn1 -- hip_rotation_l/RConn1
  vas_int_l_vas_int_l_P4_frame_fix/LConn1 -- vas_int_l_vas_int_l_P4_vas_int_l_vas_int_l_P4_y_f/RConn1
  vas_int_r_vas_int_r_P3/LConn1 -- vas_int_r_vas_int_r_P3_frame_fix/RConn1
  vas_int_r_vas_int_r_P3_vas_int_r_vas_int_r_P3_y_f/LConn1 -- vas_int_r_vas_int_r_P3_y/RConn1
  vas_int_r_vas_int_r_P3_vas_int_r_vas_int_r_P3_y_f/RConn1 -- vas_int_r_vas_int_r_P3_z/LConn1
  vas_int_r_vas_int_r_P3_vas_int_r_vas_int_r_P3_z_f/LConn1 -- vas_int_r_vas_int_r_P3_z/RConn1
  vas_int_r_vas_int_r_P3_frame_fix/LConn1 -- vas_int_r_vas_int_r_P3_vas_int_r_vas_int_r_P3_z_f/RConn1
  vas_int_r_vas_int_r_P4/LConn1 -- vas_int_r_vas_int_r_P4_frame_fix/RConn1
  vas_int_r_vas_int_r_P4_vas_int_r_vas_int_r_P4_x_f/LConn1 -- vas_int_r_vas_int_r_P4_x/RConn1
  vas_int_r_vas_int_r_P4_vas_int_r_vas_int_r_P4_x_f/RConn1 -- vas_int_r_vas_int_r_P4_y/LConn1
  vas_int_r_vas_int_r_P4_vas_int_r_vas_int_r_P4_y_f/LConn1 -- vas_int_r_vas_int_r_P4_y/RConn1
  femur_l_frame_fix/LConn1 -- femur_l_hip_rotation_l_f/RConn1
  vas_int_r_vas_int_r_P4_frame_fix/LConn1 -- vas_int_r_vas_int_r_P4_vas_int_r_vas_int_r_P4_y_f/RConn1
  vas_lat_l_vas_lat_l_P3/LConn1 -- vas_lat_l_vas_lat_l_P3_frame_fix/RConn1
  vas_lat_l_vas_lat_l_P3_vas_lat_l_vas_lat_l_P3_x_f/LConn1 -- vas_lat_l_vas_lat_l_P3_x/RConn1
  vas_lat_l_vas_lat_l_P3_vas_lat_l_vas_lat_l_P3_x_f/RConn1 -- vas_lat_l_vas_lat_l_P3_y/LConn1
  vas_lat_l_vas_lat_l_P3_vas_lat_l_vas_lat_l_P3_y_f/LConn1 -- vas_lat_l_vas_lat_l_P3_y/RConn1
  vas_lat_l_vas_lat_l_P3_vas_lat_l_vas_lat_l_P3_y_f/RConn1 -- vas_lat_l_vas_lat_l_P3_z/LConn1
  vas_lat_l_vas_lat_l_P3_vas_lat_l_vas_lat_l_P3_z_f/LConn1 -- vas_lat_l_vas_lat_l_P3_z/RConn1
  vas_lat_l_vas_lat_l_P3_frame_fix/LConn1 -- vas_lat_l_vas_lat_l_P3_vas_lat_l_vas_lat_l_P3_z_f/RConn1
  vas_lat_l_vas_lat_l_P4/LConn1 -- vas_lat_l_vas_lat_l_P4_frame_fix/RConn1
  vas_lat_l_vas_lat_l_P4_vas_lat_l_vas_lat_l_P4_x_f/LConn1 -- vas_lat_l_vas_lat_l_P4_x/RConn1
  femur_r/LConn1 -- femur_r_frame_fix/RConn1
  vas_lat_l_vas_lat_l_P4_vas_lat_l_vas_lat_l_P4_x_f/RConn1 -- vas_lat_l_vas_lat_l_P4_y/LConn1
  vas_lat_l_vas_lat_l_P4_vas_lat_l_vas_lat_l_P4_y_f/LConn1 -- vas_lat_l_vas_lat_l_P4_y/RConn1
  vas_lat_l_vas_lat_l_P4_vas_lat_l_vas_lat_l_P4_y_f/RConn1 -- vas_lat_l_vas_lat_l_P4_z/LConn1
  vas_lat_l_vas_lat_l_P4_vas_lat_l_vas_lat_l_P4_z_f/LConn1 -- vas_lat_l_vas_lat_l_P4_z/RConn1
  vas_lat_l_vas_lat_l_P4_frame_fix/LConn1 -- vas_lat_l_vas_lat_l_P4_vas_lat_l_vas_lat_l_P4_z_f/RConn1
  vas_lat_l_vas_lat_l_P5/LConn1 -- vas_lat_l_vas_lat_l_P5_frame_fix/RConn1
  vas_lat_l_vas_lat_l_P5_vas_lat_l_vas_lat_l_P5_x_f/LConn1 -- vas_lat_l_vas_lat_l_P5_x/RConn1
  vas_lat_l_vas_lat_l_P5_vas_lat_l_vas_lat_l_P5_x_f/RConn1 -- vas_lat_l_vas_lat_l_P5_y/LConn1
  vas_lat_l_vas_lat_l_P5_vas_lat_l_vas_lat_l_P5_y_f/LConn1 -- vas_lat_l_vas_lat_l_P5_y/RConn1
  vas_lat_l_vas_lat_l_P5_frame_fix/LConn1 -- vas_lat_l_vas_lat_l_P5_vas_lat_l_vas_lat_l_P5_y_f/RConn1
  femur_r/RConn8 -- knee_r_translation1/LConn1
  vas_lat_r_vas_lat_r_P3/LConn1 -- vas_lat_r_vas_lat_r_P3_frame_fix/RConn1
  vas_lat_r_vas_lat_r_P3_vas_lat_r_vas_lat_r_P3_x_f/LConn1 -- vas_lat_r_vas_lat_r_P3_x/RConn1
  vas_lat_r_vas_lat_r_P3_vas_lat_r_vas_lat_r_P3_x_f/RConn1 -- vas_lat_r_vas_lat_r_P3_y/LConn1
  vas_lat_r_vas_lat_r_P3_vas_lat_r_vas_lat_r_P3_y_f/LConn1 -- vas_lat_r_vas_lat_r_P3_y/RConn1
  vas_lat_r_vas_lat_r_P3_vas_lat_r_vas_lat_r_P3_y_f/RConn1 -- vas_lat_r_vas_lat_r_P3_z/LConn1
  vas_lat_r_vas_lat_r_P3_vas_lat_r_vas_lat_r_P3_z_f/LConn1 -- vas_lat_r_vas_lat_r_P3_z/RConn1
  vas_lat_r_vas_lat_r_P3_frame_fix/LConn1 -- vas_lat_r_vas_lat_r_P3_vas_lat_r_vas_lat_r_P3_z_f/RConn1
  vas_lat_r_vas_lat_r_P4/LConn1 -- vas_lat_r_vas_lat_r_P4_frame_fix/RConn1
  vas_lat_r_vas_lat_r_P4_vas_lat_r_vas_lat_r_P4_x_f/LConn1 -- vas_lat_r_vas_lat_r_P4_x/RConn1
  vas_lat_r_vas_lat_r_P4_vas_lat_r_vas_lat_r_P4_x_f/RConn1 -- vas_lat_r_vas_lat_r_P4_y/LConn1
  femur_r/RConn7 -- lat_gas_r_lat_gas_r_P2_x/LConn1
  vas_lat_r_vas_lat_r_P4_vas_lat_r_vas_lat_r_P4_y_f/LConn1 -- vas_lat_r_vas_lat_r_P4_y/RConn1
  vas_lat_r_vas_lat_r_P4_vas_lat_r_vas_lat_r_P4_y_f/RConn1 -- vas_lat_r_vas_lat_r_P4_z/LConn1
  vas_lat_r_vas_lat_r_P4_vas_lat_r_vas_lat_r_P4_z_f/LConn1 -- vas_lat_r_vas_lat_r_P4_z/RConn1
  vas_lat_r_vas_lat_r_P4_frame_fix/LConn1 -- vas_lat_r_vas_lat_r_P4_vas_lat_r_vas_lat_r_P4_z_f/RConn1
  vas_lat_r_vas_lat_r_P5/LConn1 -- vas_lat_r_vas_lat_r_P5_frame_fix/RConn1
  vas_lat_r_vas_lat_r_P5_vas_lat_r_vas_lat_r_P5_x_f/LConn1 -- vas_lat_r_vas_lat_r_P5_x/RConn1
  vas_lat_r_vas_lat_r_P5_vas_lat_r_vas_lat_r_P5_x_f/RConn1 -- vas_lat_r_vas_lat_r_P5_y/LConn1
  vas_lat_r_vas_lat_r_P5_vas_lat_r_vas_lat_r_P5_y_f/LConn1 -- vas_lat_r_vas_lat_r_P5_y/RConn1
  vas_lat_r_vas_lat_r_P5_frame_fix/LConn1 -- vas_lat_r_vas_lat_r_P5_vas_lat_r_vas_lat_r_P5_y_f/RConn1
  vas_med_l_vas_med_l_P3/LConn1 -- vas_med_l_vas_med_l_P3_frame_fix/RConn1
  femur_r/RConn6 -- med_gas_r_med_gas_r_P2_x/LConn1
  vas_med_l_vas_med_l_P3_vas_med_l_vas_med_l_P3_x_f/LConn1 -- vas_med_l_vas_med_l_P3_x/RConn1
  vas_med_l_vas_med_l_P3_vas_med_l_vas_med_l_P3_x_f/RConn1 -- vas_med_l_vas_med_l_P3_y/LConn1
  vas_med_l_vas_med_l_P3_vas_med_l_vas_med_l_P3_y_f/LConn1 -- vas_med_l_vas_med_l_P3_y/RConn1
  vas_med_l_vas_med_l_P3_vas_med_l_vas_med_l_P3_y_f/RConn1 -- vas_med_l_vas_med_l_P3_z/LConn1
  vas_med_l_vas_med_l_P3_vas_med_l_vas_med_l_P3_z_f/LConn1 -- vas_med_l_vas_med_l_P3_z/RConn1
  vas_med_l_vas_med_l_P3_frame_fix/LConn1 -- vas_med_l_vas_med_l_P3_vas_med_l_vas_med_l_P3_z_f/RConn1
  vas_med_l_vas_med_l_P4/LConn1 -- vas_med_l_vas_med_l_P4_frame_fix/RConn1
  vas_med_l_vas_med_l_P4_vas_med_l_vas_med_l_P4_x_f/LConn1 -- vas_med_l_vas_med_l_P4_x/RConn1
  vas_med_l_vas_med_l_P4_vas_med_l_vas_med_l_P4_x_f/RConn1 -- vas_med_l_vas_med_l_P4_y/LConn1
  vas_med_l_vas_med_l_P4_vas_med_l_vas_med_l_P4_y_f/LConn1 -- vas_med_l_vas_med_l_P4_y/RConn1
  femur_r/RConn5 -- vas_int_r_vas_int_r_P3_y/LConn1
  vas_med_l_vas_med_l_P4_vas_med_l_vas_med_l_P4_y_f/RConn1 -- vas_med_l_vas_med_l_P4_z/LConn1
  vas_med_l_vas_med_l_P4_vas_med_l_vas_med_l_P4_z_f/LConn1 -- vas_med_l_vas_med_l_P4_z/RConn1
  vas_med_l_vas_med_l_P4_frame_fix/LConn1 -- vas_med_l_vas_med_l_P4_vas_med_l_vas_med_l_P4_z_f/RConn1
  vas_med_l_vas_med_l_P5/LConn1 -- vas_med_l_vas_med_l_P5_frame_fix/RConn1
  vas_med_l_vas_med_l_P5_vas_med_l_vas_med_l_P5_x_f/LConn1 -- vas_med_l_vas_med_l_P5_x/RConn1
  vas_med_l_vas_med_l_P5_vas_med_l_vas_med_l_P5_x_f/RConn1 -- vas_med_l_vas_med_l_P5_y/LConn1
  vas_med_l_vas_med_l_P5_vas_med_l_vas_med_l_P5_y_f/LConn1 -- vas_med_l_vas_med_l_P5_y/RConn1
  vas_med_l_vas_med_l_P5_frame_fix/LConn1 -- vas_med_l_vas_med_l_P5_vas_med_l_vas_med_l_P5_y_f/RConn1
  vas_med_r_vas_med_r_P3/LConn1 -- vas_med_r_vas_med_r_P3_frame_fix/RConn1
  vas_med_r_vas_med_r_P3_vas_med_r_vas_med_r_P3_x_f/LConn1 -- vas_med_r_vas_med_r_P3_x/RConn1
  femur_r/RConn4 -- vas_lat_r_vas_lat_r_P3_x/LConn1
  vas_med_r_vas_med_r_P3_vas_med_r_vas_med_r_P3_x_f/RConn1 -- vas_med_r_vas_med_r_P3_y/LConn1
  vas_med_r_vas_med_r_P3_vas_med_r_vas_med_r_P3_y_f/LConn1 -- vas_med_r_vas_med_r_P3_y/RConn1
  vas_med_r_vas_med_r_P3_vas_med_r_vas_med_r_P3_y_f/RConn1 -- vas_med_r_vas_med_r_P3_z/LConn1
  vas_med_r_vas_med_r_P3_vas_med_r_vas_med_r_P3_z_f/LConn1 -- vas_med_r_vas_med_r_P3_z/RConn1
  vas_med_r_vas_med_r_P3_frame_fix/LConn1 -- vas_med_r_vas_med_r_P3_vas_med_r_vas_med_r_P3_z_f/RConn1
  vas_med_r_vas_med_r_P4/LConn1 -- vas_med_r_vas_med_r_P4_frame_fix/RConn1
  vas_med_r_vas_med_r_P4_vas_med_r_vas_med_r_P4_x_f/LConn1 -- vas_med_r_vas_med_r_P4_x/RConn1
  vas_med_r_vas_med_r_P4_vas_med_r_vas_med_r_P4_x_f/RConn1 -- vas_med_r_vas_med_r_P4_y/LConn1
  vas_med_r_vas_med_r_P4_vas_med_r_vas_med_r_P4_y_f/LConn1 -- vas_med_r_vas_med_r_P4_y/RConn1
  vas_med_r_vas_med_r_P4_vas_med_r_vas_med_r_P4_y_f/RConn1 -- vas_med_r_vas_med_r_P4_z/LConn1
  femur_r/RConn3 -- vas_lat_r_vas_lat_r_P4_x/LConn1
  vas_med_r_vas_med_r_P4_vas_med_r_vas_med_r_P4_z_f/LConn1 -- vas_med_r_vas_med_r_P4_z/RConn1
  vas_med_r_vas_med_r_P4_frame_fix/LConn1 -- vas_med_r_vas_med_r_P4_vas_med_r_vas_med_r_P4_z_f/RConn1
  vas_med_r_vas_med_r_P5/LConn1 -- vas_med_r_vas_med_r_P5_frame_fix/RConn1
  vas_med_r_vas_med_r_P5_vas_med_r_vas_med_r_P5_x_f/LConn1 -- vas_med_r_vas_med_r_P5_x/RConn1
  vas_med_r_vas_med_r_P5_vas_med_r_vas_med_r_P5_x_f/RConn1 -- vas_med_r_vas_med_r_P5_y/LConn1
  vas_med_r_vas_med_r_P5_vas_med_r_vas_med_r_P5_y_f/LConn1 -- vas_med_r_vas_med_r_P5_y/RConn1
  vas_med_r_vas_med_r_P5_frame_fix/LConn1 -- vas_med_r_vas_med_r_P5_vas_med_r_vas_med_r_P5_y_f/RConn1
  pelvis_tx/LConn1 -- world/RConn1
  World/RConn1 -- MechanismConfiguration/RConn1 -- Solver Configuration/RConn1 -- world/LConn1
  calcn_l_frame_fix/LConn1 -- calcn_l_subtalar_angle_l_f/RConn1
  femur_r/RConn2 -- vas_med_r_vas_med_r_P3_x/LConn1
  femur_r/RConn1 -- vas_med_r_vas_med_r_P4_x/LConn1
  femur_r_hip_adduction_r_f/LConn1 -- hip_adduction_r/RConn1
  femur_r_hip_adduction_r_f/RConn1 -- hip_rotation_r/LConn1
  femur_r_hip_flexion_r_f/LConn1 -- hip_flexion_r/RConn1
  femur_r_hip_flexion_r_f/RConn1 -- hip_adduction_r/LConn1
  femur_r_hip_rotation_r_f/LConn1 -- hip_rotation_r/RConn1
  femur_r_frame_fix/LConn1 -- femur_r_hip_rotation_r_f/RConn1
  grac_l_grac_l_P2/LConn1 -- grac_l_grac_l_P2_frame_fix/RConn1
  grac_l_grac_l_P2_grac_l_grac_l_P2_x_f/LConn1 -- grac_l_grac_l_P2_x/RConn1
  calcn_r/LConn1 -- calcn_r_frame_fix/RConn1
  grac_l_grac_l_P2_grac_l_grac_l_P2_x_f/RConn1 -- grac_l_grac_l_P2_y/LConn1
  grac_l_grac_l_P2_grac_l_grac_l_P2_y_f/LConn1 -- grac_l_grac_l_P2_y/RConn1
  grac_l_grac_l_P2_grac_l_grac_l_P2_y_f/RConn1 -- grac_l_grac_l_P2_z/LConn1
  grac_l_grac_l_P2_grac_l_grac_l_P2_z_f/LConn1 -- grac_l_grac_l_P2_z/RConn1
  grac_l_grac_l_P2_frame_fix/LConn1 -- grac_l_grac_l_P2_grac_l_grac_l_P2_z_f/RConn1
  grac_r_grac_r_P2/LConn1 -- grac_r_grac_r_P2_frame_fix/RConn1
  grac_r_grac_r_P2_grac_r_grac_r_P2_x_f/LConn1 -- grac_r_grac_r_P2_x/RConn1
  grac_r_grac_r_P2_grac_r_grac_r_P2_x_f/RConn1 -- grac_r_grac_r_P2_y/LConn1
  grac_r_grac_r_P2_grac_r_grac_r_P2_y_f/LConn1 -- grac_r_grac_r_P2_y/RConn1
  grac_r_grac_r_P2_grac_r_grac_r_P2_y_f/RConn1 -- grac_r_grac_r_P2_z/LConn1
  calcn_r/RConn1 -- mtp_angle_r/LConn1
  grac_r_grac_r_P2_grac_r_grac_r_P2_z_f/LConn1 -- grac_r_grac_r_P2_z/RConn1
  grac_r_grac_r_P2_frame_fix/LConn1 -- grac_r_grac_r_P2_grac_r_grac_r_P2_z_f/RConn1
  iliacus_l_iliacus_l_P3/LConn1 -- iliacus_l_iliacus_l_P3_frame_fix/RConn1
  iliacus_l_iliacus_l_P3_iliacus_l_iliacus_l_P3_x_f/LConn1 -- iliacus_l_iliacus_l_P3_x/RConn1
  iliacus_l_iliacus_l_P3_iliacus_l_iliacus_l_P3_x_f/RConn1 -- iliacus_l_iliacus_l_P3_y/LConn1
  iliacus_l_iliacus_l_P3_iliacus_l_iliacus_l_P3_y_f/LConn1 -- iliacus_l_iliacus_l_P3_y/RConn1
  iliacus_l_iliacus_l_P3_frame_fix/LConn1 -- iliacus_l_iliacus_l_P3_iliacus_l_iliacus_l_P3_y_f/RConn1
  iliacus_r_iliacus_r_P3/LConn1 -- iliacus_r_iliacus_r_P3_frame_fix/RConn1
  iliacus_r_iliacus_r_P3_iliacus_r_iliacus_r_P3_x_f/LConn1 -- iliacus_r_iliacus_r_P3_x/RConn1
  iliacus_r_iliacus_r_P3_iliacus_r_iliacus_r_P3_x_f/RConn1 -- iliacus_r_iliacus_r_P3_y/LConn1
  calcn_r_subtalar_angle_r_f/LConn1 -- subtalar_angle_r/RConn1
  iliacus_r_iliacus_r_P3_iliacus_r_iliacus_r_P3_y_f/LConn1 -- iliacus_r_iliacus_r_P3_y/RConn1
  iliacus_r_iliacus_r_P3_frame_fix/LConn1 -- iliacus_r_iliacus_r_P3_iliacus_r_iliacus_r_P3_y_f/RConn1
  lat_gas_l_lat_gas_l_P2/LConn1 -- lat_gas_l_lat_gas_l_P2_frame_fix/RConn1
  lat_gas_l_lat_gas_l_P2_lat_gas_l_lat_gas_l_P2_x_f/LConn1 -- lat_gas_l_lat_gas_l_P2_x/RConn1
  lat_gas_l_lat_gas_l_P2_lat_gas_l_lat_gas_l_P2_x_f/RConn1 -- lat_gas_l_lat_gas_l_P2_y/LConn1
  lat_gas_l_lat_gas_l_P2_lat_gas_l_lat_gas_l_P2_y_f/LConn1 -- lat_gas_l_lat_gas_l_P2_y/RConn1
  lat_gas_l_lat_gas_l_P2_frame_fix/LConn1 -- lat_gas_l_lat_gas_l_P2_lat_gas_l_lat_gas_l_P2_y_f/RConn1
  lat_gas_r_lat_gas_r_P2/LConn1 -- lat_gas_r_lat_gas_r_P2_frame_fix/RConn1
  lat_gas_r_lat_gas_r_P2_lat_gas_r_lat_gas_r_P2_x_f/LConn1 -- lat_gas_r_lat_gas_r_P2_x/RConn1
  lat_gas_r_lat_gas_r_P2_lat_gas_r_lat_gas_r_P2_x_f/RConn1 -- lat_gas_r_lat_gas_r_P2_y/LConn1
  calcn_r_frame_fix/LConn1 -- calcn_r_subtalar_angle_r_f/RConn1
  lat_gas_r_lat_gas_r_P2_lat_gas_r_lat_gas_r_P2_y_f/LConn1 -- lat_gas_r_lat_gas_r_P2_y/RConn1
  lat_gas_r_lat_gas_r_P2_frame_fix/LConn1 -- lat_gas_r_lat_gas_r_P2_lat_gas_r_lat_gas_r_P2_y_f/RConn1
  med_gas_l_med_gas_l_P2/LConn1 -- med_gas_l_med_gas_l_P2_frame_fix/RConn1
  med_gas_l_med_gas_l_P2_med_gas_l_med_gas_l_P2_x_f/LConn1 -- med_gas_l_med_gas_l_P2_x/RConn1
  med_gas_l_med_gas_l_P2_med_gas_l_med_gas_l_P2_x_f/RConn1 -- med_gas_l_med_gas_l_P2_y/LConn1
  med_gas_l_med_gas_l_P2_med_gas_l_med_gas_l_P2_y_f/LConn1 -- med_gas_l_med_gas_l_P2_y/RConn1
  med_gas_l_med_gas_l_P2_med_gas_l_med_gas_l_P2_y_f/RConn1 -- med_gas_l_med_gas_l_P2_z/LConn1
  med_gas_l_med_gas_l_P2_med_gas_l_med_gas_l_P2_z_f/LConn1 -- med_gas_l_med_gas_l_P2_z/RConn1
  med_gas_l_med_gas_l_P2_frame_fix/LConn1 -- med_gas_l_med_gas_l_P2_med_gas_l_med_gas_l_P2_z_f/RConn1
  med_gas_r_med_gas_r_P2/LConn1 -- med_gas_r_med_gas_r_P2_frame_fix/RConn1
  femur_l/LConn1 -- femur_l_frame_fix/RConn1
  med_gas_r_med_gas_r_P2_med_gas_r_med_gas_r_P2_x_f/LConn1 -- med_gas_r_med_gas_r_P2_x/RConn1
  med_gas_r_med_gas_r_P2_med_gas_r_med_gas_r_P2_x_f/RConn1 -- med_gas_r_med_gas_r_P2_y/LConn1
  med_gas_r_med_gas_r_P2_med_gas_r_med_gas_r_P2_y_f/LConn1 -- med_gas_r_med_gas_r_P2_y/RConn1
  med_gas_r_med_gas_r_P2_med_gas_r_med_gas_r_P2_y_f/RConn1 -- med_gas_r_med_gas_r_P2_z/LConn1
  med_gas_r_med_gas_r_P2_med_gas_r_med_gas_r_P2_z_f/LConn1 -- med_gas_r_med_gas_r_P2_z/RConn1
  med_gas_r_med_gas_r_P2_frame_fix/LConn1 -- med_gas_r_med_gas_r_P2_med_gas_r_med_gas_r_P2_z_f/RConn1
  pelvis/LConn1 -- pelvis_frame_fix/RConn1
  hip_flexion_l/LConn1 -- pelvis/RConn7
  hip_flexion_r/LConn1 -- pelvis/RConn6
  iliacus_l_iliacus_l_P3_x/LConn1 -- pelvis/RConn5
  femur_l/RConn8 -- knee_l_translation1/LConn1
  iliacus_r_iliacus_r_P3_x/LConn1 -- pelvis/RConn4
  lumbar_extension/LConn1 -- pelvis/RConn3
  pelvis/RConn2 -- psoas_l_psoas_l_P3_x/LConn1
  pelvis/RConn1 -- psoas_r_psoas_r_P3_x/LConn1
  pelvis_list/RConn1 -- pelvis_pelvis_list_f/LConn1
  pelvis_pelvis_list_f/RConn1 -- pelvis_rotation/LConn1
  pelvis_pelvis_rotation_f/LConn1 -- pelvis_rotation/RConn1
  pelvis_frame_fix/LConn1 -- pelvis_pelvis_rotation_f/RConn1
  pelvis_pelvis_tilt_f/LConn1 -- pelvis_tilt/RConn1
  pelvis_list/LConn1 -- pelvis_pelvis_tilt_f/RConn1
